simulink model "three_phase_cycloconverter"  (R2024a)
settings: Solver=VariableStepAuto  StartTime=0.0  StopTime=0.2  MaxStep=1e-4  RelTol=1e-3
undefined symbols (not defined in the file): D
libraries: spsThyristorLib x12, spsACVoltageSourceLib x3, spsGroundLib x2, spsIdealSwitchLib x2, spsVoltageMeasurementLib x1, spsRMSLib x1, spsSeriesRLCBranchLib x1, spspowerguiLib x1
settings Model: Creator=Asus  LastModifiedBy=Asus
settings DebuggingCC: UnconnectedInputMsg=warning  UnconnectedOutputMsg=warning  UnconnectedLineMsg=warning
settings ModelReferenceCC: EnableRefExpFcnMdlSchedulingChecks=on
settings RTWCC: GPUComputeCapability=3.5  DLArmComputeVersion=19.05

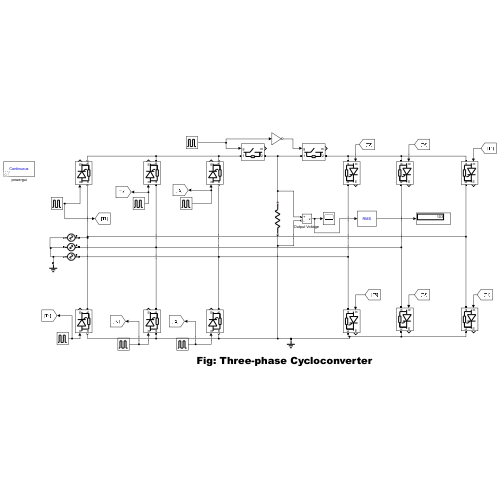
[thumbnail: Simulink's stored preview of the top-level diagram]
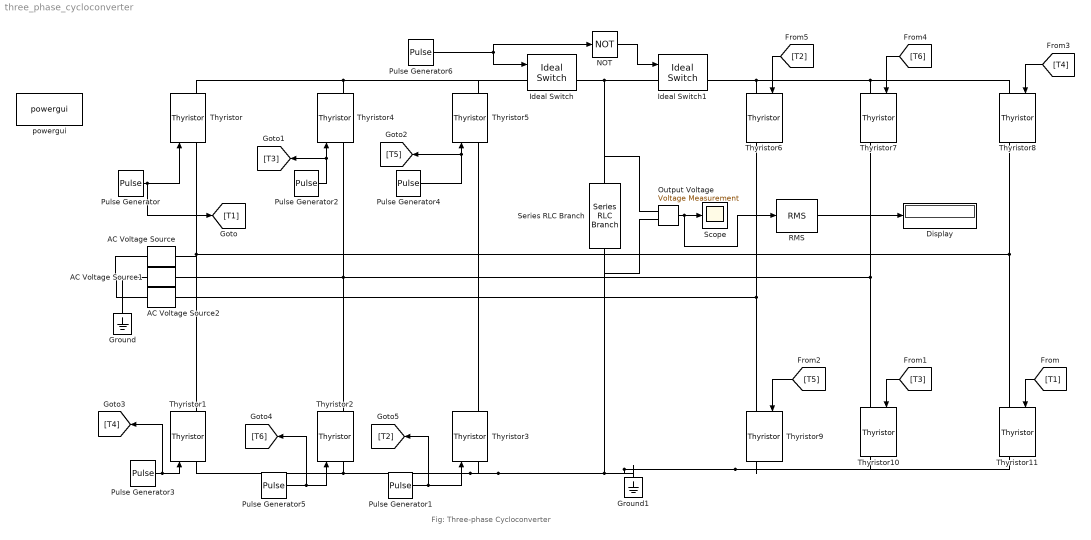
== system three_phase_cycloconverter ==
  note: Fig: Three-phase Cycloconverter
  AC Voltage Source : spsACVoltageSourceLib/AC Voltage Source  Amplitude=120  Phase=0  Frequency=50  SampleTime=0  Measurements=None  BusType=swing  Pref=10e3  Qref=0  Qmin=-inf  Qmax=+inf
  AC Voltage Source1 : spsACVoltageSourceLib/AC Voltage Source  Amplitude=120  Phase=-120  Frequency=50  SampleTime=0  Measurements=None  BusType=swing  Pref=10e3  Qref=0  Qmin=-inf  Qmax=+inf
  AC Voltage Source2 : spsACVoltageSourceLib/AC Voltage Source  Amplitude=120  Phase=120  Frequency=50  SampleTime=0  Measurements=None  BusType=swing  Pref=10e3  Qref=0  Qmin=-inf  Qmax=+inf
  Display : Display
  Ground : spsGroundLib/Ground  LConnTagsString=a
  Ground1 : spsGroundLib/Ground  LConnTagsString=a
  Ideal Switch : spsIdealSwitchLib/Ideal Switch  Ron=0.001  Lon=0  IC=0  Rs=1e5  Cs=inf  Measurements=on
  Ideal Switch1 : spsIdealSwitchLib/Ideal Switch  Ron=0.001  Lon=0  IC=0  Rs=1e5  Cs=inf  Measurements=on
  NOT : Logic  Operator=NOT  IconShape=distinctive  AllPortsSameDT=off  OutDataTypeStr=boolean
  "Output Voltage " : spsVoltageMeasurementLib/Voltage Measurement  PhasorSimulation=off  OutputType=Complex  PSBequivalent=0
  Pulse Generator : DiscretePulseGenerator  PulseType=Time based  Amplitude=10  Period=1/50  PulseWidth=10  PhaseDelay=(1/50)*(30+D)/360
  Pulse Generator1 : DiscretePulseGenerator  PulseType=Time based  Amplitude=10  Period=1/50  PulseWidth=10  PhaseDelay=(1/50)*(90+D)/360
  Pulse Generator2 : DiscretePulseGenerator  PulseType=Time based  Amplitude=10  Period=1/50  PulseWidth=10  PhaseDelay=(1/50)*(150+D)/360
  Pulse Generator3 : DiscretePulseGenerator  PulseType=Time based  Amplitude=10  Period=1/50  PulseWidth=10  PhaseDelay=(1/50)*(210+D)/360
  Pulse Generator4 : DiscretePulseGenerator  PulseType=Time based  Amplitude=10  Period=1/50  PulseWidth=10  PhaseDelay=(1/50)*(270+D)/360
  Pulse Generator5 : DiscretePulseGenerator  PulseType=Time based  Amplitude=10  Period=1/50  PulseWidth=10  PhaseDelay=(1/50)*(330+D)/360
  Pulse Generator6 : DiscretePulseGenerator  PulseType=Time based  Amplitude=10  Period=3/50  PulseWidth=50
  RMS : spsRMSLib/RMS  TrueRMS=on  Freq=60  RMSInit=120  Ts=0
  Scope : Scope
  Series RLC Branch : spsSeriesRLCBranchLib/Series RLC Branch  LConnTagsString=__new0  RConnTagsString=__new0  BranchType=R  Resistance=5  Inductance=1e-3  SetiL0=off  InitialCurrent=0  Capacitance=1e-6  Setx0=off  InitialVoltage=0  Measurements=None
  Thyristor{,1..11} (12 alike) : spsThyristorLib/Thyristor  Ron=0.001  Lon=0  Vf=0.8  IC=0  Rs=500  Cs=250e-9  Measurements=on
  powergui : spspowerguiLib/powergui  Priority=1  SimulationMode=Continuous  SampleTime=50e-6  frequency=60  Iterations=50  frequencyindice=50  Pbase=100e6  ErrMax=1e-4  UnitsV=kV  UnitsW=MW  buscounter=0  FunctionMessages=off  echomessages=off  EnableUseOfTLC=off  CurrentSourceSwitches=off  DisableSnubberDevices=off  DisableRonSwitches=off  DisableVfSwitches=off  DisplayEquations=off  AutomaticDiscreteSolvers=off  SolverType=Tustin/Backward Euler (TBE)  Interpol=off  ExternalGateDelay=off  methode=off  Ts=100  x0status=blocks  SPID=on  SwTol=0  HookPort=off  NonlinearTolerance=1e-4  nMaxIteration=100  ContinueOnMaxIteration=off  RestoreLinks=warning  ResistiveCurrentMeasurement=off  Frange=[0:2:500]  Ylog=off  Xlog=on  ShowGrid=off  save=off  variable=ZData  structure=0  ZoomFFT=off  StartTime=0.0  cycles=1  DisplayStyle=1  fundamental=60  FreqAxis=off  MaxFrequency=1000  frequencyindicesteady=1  RmsSteady=1  display=off
  wires:
  "Output Voltage "/1 -> RMS/1, Scope/1
  Pulse Generator/1 -> [T1], Thyristor/1
  Pulse Generator1/1 -> [T2], Thyristor3/1
  Pulse Generator2/1 -> [T3], Thyristor4/1
  Pulse Generator3/1 -> [T4], Thyristor1/1
  Pulse Generator4/1 -> [T5], Thyristor5/1
  Pulse Generator5/1 -> [T6], Thyristor2/1
  Pulse Generator6/1 -> Ideal Switch/1, NOT/1
  NOT/1 -> Ideal Switch1/1
  [T1] -> Thyristor11/1
  [T3] -> Thyristor10/1
  [T5] -> Thyristor9/1
  [T4] -> Thyristor8/1
  [T6] -> Thyristor7/1
  [T2] -> Thyristor6/1
  RMS/1 -> Display/1
  connections:
  Thyristor/RConn1 -- Ideal Switch/LConn1 -- Thyristor5/RConn1 -- Thyristor4/RConn1
  Thyristor7/RConn1 -- Thyristor4/LConn1 -- Thyristor2/RConn1 -- AC Voltage Source1/RConn1 -- Thyristor10/LConn1
  Thyristor6/LConn1 -- Ideal Switch1/RConn1 -- Thyristor8/LConn1 -- Thyristor7/LConn1
  Thyristor1/LConn1 -- "Output Voltage "/LConn2 -- Series RLC Branch/RConn1 -- Thyristor11/RConn1 -- Thyristor10/RConn1 -- Thyristor9/RConn1 -- Ground1/LConn1 -- Thyristor3/LConn1 -- Thyristor2/LConn1
  Ideal Switch1/LConn1 -- "Output Voltage "/LConn1 -- Series RLC Branch/LConn1 -- Ideal Switch/RConn1
  AC Voltage Source/LConn1 -- AC Voltage Source2/LConn1 -- Ground/LConn1 -- AC Voltage Source1/LConn1
  Thyristor8/RConn1 -- Thyristor/LConn1 -- Thyristor1/RConn1 -- AC Voltage Source/RConn1 -- Thyristor11/LConn1
  Thyristor9/LConn1 -- Thyristor3/RConn1 -- Thyristor5/LConn1 -- AC Voltage Source2/RConn1 -- Thyristor6/RConn1
